simulink model "bicyclemodel_step"  (R2020b)
settings: Solver=ode5  StartTime=0.0  StopTime=tf  FixedStep=dt  RelTol=1e-3
values from neighbouring files (symbols this model uses):
  I = 2500    [bicyclemodle_setp_disturbance_force_Param.m]    (also in bicyclemodle_stepParam.m; twoDOFmodel_side_wind_gust_Param.m)
  Kf = 55000    [bicyclemodle_setp_disturbance_force_Param.m]    (also in bicyclemodle_stepParam.m; twoDOFmodel_side_wind_gust_Param.m)
  lf = 1.1    [bicyclemodle_setp_disturbance_force_Param.m]    (also in bicyclemodle_stepParam.m; twoDOFmodel_side_wind_gust_Param.m)
  m = 1500    [bicyclemodle_setp_disturbance_force_Param.m]    (also in bicyclemodle_stepParam.m; twoDOFmodel_side_wind_gust_Param.m)
  Sf = 0.0    (= 0)    [bicyclemodle_setp_disturbance_force_Param.m]    (also in bicyclemodle_stepParam.m = 0.04; twoDOFmodel_side_wind_gust_Param.m)
  V = 80/3.6    (= 22.2222222222)    [bicyclemodle_setp_disturbance_force_Param.m]    (also in bicyclemodle_stepParam.m = 38.8888888889; twoDOFmodel_side_wind_gust_Param.m = 40)
settings Model: Creator=Anson  LastModifiedBy=Anson

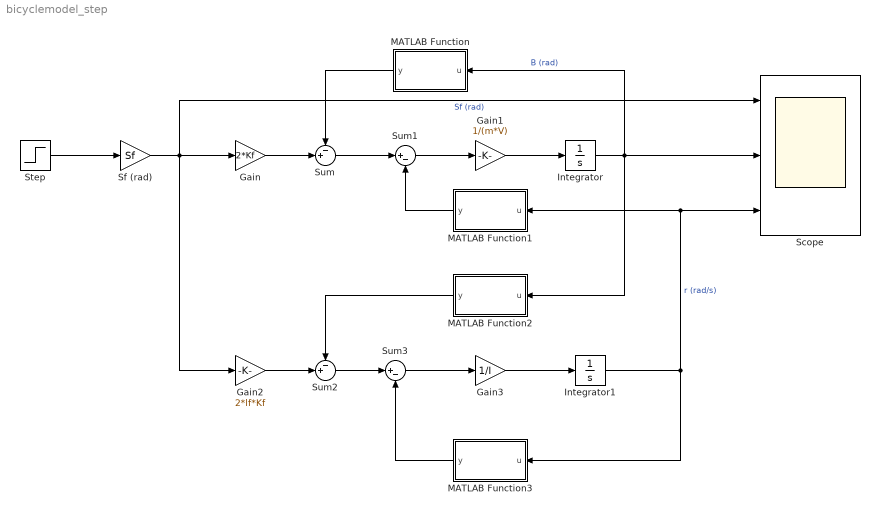
== system bicyclemodel_step ==
  Gain : Gain  Gain=2*Kf
  Gain1 : Gain  Gain=1/(m*V)
  Gain2 : Gain  Gain=2*lf*Kf
  Gain3 : Gain  Gain=1/I
  Integrator : Integrator
  Integrator1 : Integrator
  MATLAB Function : MATLAB Function  TreatAsAtomicUnit=on
  MATLAB Function1 : MATLAB Function  TreatAsAtomicUnit=on
  MATLAB Function2 : MATLAB Function  TreatAsAtomicUnit=on
  MATLAB Function3 : MATLAB Function  TreatAsAtomicUnit=on
  Scope : Scope  NumInputPorts=3
  Sf (rad) : Gain  Gain=Sf
  Step : Step  SampleTime=0
  Sum : Sum  Inputs=-+|
  Sum1 : Sum  Inputs=|+-
  Sum2 : Sum  Inputs=-+|
  Sum3 : Sum  Inputs=|+-
  wires:
  Step/1 -> Sf (rad)/1
  Sf (rad)/1 -> Gain2/1, Scope/1, Gain/1  "Sf (rad)"
  Gain/1 -> Sum/2
  Sum/1 -> Sum1/1
  Sum1/1 -> Gain1/1
  Gain1/1 -> Integrator/1
  Integrator/1 -> MATLAB Function2/1(u), MATLAB Function/1(u), Scope/2  "B (rad)"
  MATLAB Function/1(y) -> Sum/1
  MATLAB Function1/1(y) -> Sum1/2
  Gain2/1 -> Sum2/2
  Sum2/1 -> Sum3/1
  Sum3/1 -> Gain3/1
  MATLAB Function2/1(y) -> Sum2/1
  Gain3/1 -> Integrator1/1
  Integrator1/1 -> MATLAB Function3/1(u), MATLAB Function1/1(u), Scope/3  "r (rad/s)"
  MATLAB Function3/1(y) -> Sum3/2

== matlab function bicyclemodel_step/MATLAB Function ==
  data: u input; y output
function y = fcn(u)
Kf = 55000; % front cornering stiffness (N/rad)
Kr = 60000; % rear cornering stiffness (N/rad)
y = 2*(Kf+Kr)*u;

== matlab function bicyclemodel_step/MATLAB Function2 ==
  data: u input; y output
function y = fcn(u)
lf = 1.1;   % distance from C.O.G to front axle (m)
lr = 1.6;   % distacne from C.O.G to rear axle (m)
Kf = 55000; % front cornering stiffness (N/rad)
Kr = 60000; % rear cornering stiffness (N/rad)
y = 2*(lf*Kf-lr*Kr)*u;

== matlab function bicyclemodel_step/MATLAB Function3 ==
  data: u input; y output
function y = fcn(u)
lf = 1.1;   % distance from C.O.G to front axle (m)
lr = 1.6;   % distacne from C.O.G to rear axle (m)
Kf = 55000; % front cornering stiffness (N/rad)
Kr = 60000; % rear cornering stiffness (N/rad)
V = 140/3.6;% velocity (m/s)
y = ((2/V)*(lf*lf*Kf+lr*lr*Kr))*u;

== matlab function bicyclemodel_step/MATLAB Function1 ==
  data: u input; y output
function y = fcn(u)
m = 1500;   % mass (kg)
lf = 1.1;   % distance from C.O.G to front axle (m)
lr = 1.6;   % distacne from C.O.G to rear axle (m)
Kf = 55000; % front cornering stiffness (N/rad)
Kr = 60000; % rear cornering stiffness (N/rad)
V = 140/3.6;% velocity (m/s)
y = (m*V+(2/V)*(lf*Kf-lr*Kr))*u;
